simulink model "calc"  (R2021a)
settings: Solver=VariableStepAuto  StartTime=0.0  StopTime=10.0  RelTol=1e-3
undefined symbols (not defined in the file or in its folder): sigbuilder_block
settings Model: Creator=tomonori  LastModifiedBy=tomonori

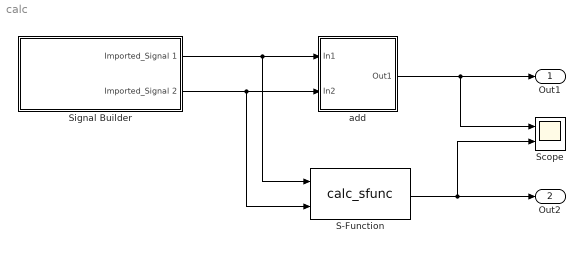
== system calc ==
  S-Function : S-Function  FunctionName=calc_sfunc  SFunctionDeploymentMode=off  EnableBusSupport=off
  Scope : Scope  NumInputPorts=2
  Signal Builder : Subsystem  Tag=STV Subsys  LoadFcn=sigbuilder_block('load',[4.5 187.5 550.5 387.75 ]);  StartFcn=sigbuilder_block('start');  StopFcn=sigbuilder_block('stop');  ClipboardFcn=sigbuilder_block('clipboard');  mask(Sigbuilder block){tuvar=[0:10]}
      mask help: Simulink:masks:SigbuilderBlock_MD
      mask init:
      | if ~strcmp(get_param(bdroot(gcbh),'SimulationStatus'),'stopped') tuvar = sigbuilder_block('maskInit'); end
      settings: CopyFcn=sigbuilder_block('copy');  DeleteFcn=sigbuilder_block('delete');  ModelCloseFcn=sigbuilder_block('modelClose');  PreSaveFcn=sigbuilder_block('preSave');  PauseFcn=sigbuilder_block('pause');  ContinueFcn=sigbuilder_block('continue');  NameChangeFcn=sigbuilder_block('namechange');  OpenFcn=sigbuilder_block('open',[4.5 187.5 550.5 387.75 ]);  CloseFcn=sigbuilder_block('close');
      mask Display: plot(0, 0, 100, 100,[2, 2, 32, 32, 2], [68, 8, 8, 68, 68],[32, 2], [38, 38], [32, 19, 2],[53, 60, 44], [32, 17, 17, 2],[16, 16, 31, 31]);txt = getActiveGroup(gcbh);text(2, 100, txt,'verticalAlignment', 'top');
  add : Subsystem
  Out1 : Outport
  Out2 : Outport  Port=2
  wires:
  Signal Builder/1(Imported_Signal 1) -> S-Function/1, add/1(In1)
  Signal Builder/2(Imported_Signal 2) -> S-Function/2, add/2(In2)
  add/1(Out1) -> Scope/1, Out1/1
  S-Function/1 -> Scope/2, Out2/1

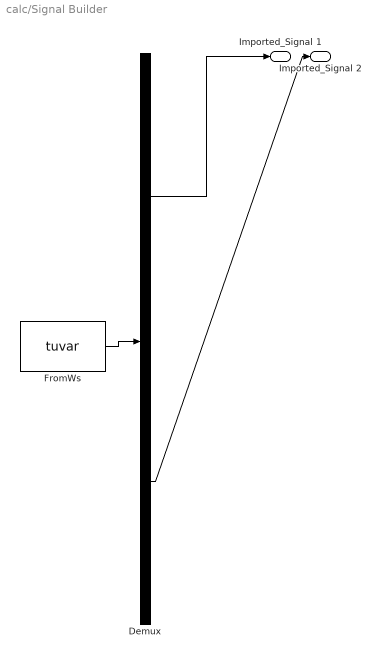
== system calc/Signal Builder ==
  Demux : Demux  Tag=STV Demux  Outputs=2
      settings: DisplayOption=none
  FromWs : FromWorkspace  Tag=STV FromWs  VariableName=tuvar
      SigBuilderData=|
      | common.afterFinalStr = 'Extrapolate'
      | common.sampleTime = 0
      | dataSet.timeRange = [1 10]
      | dataSet.name = 'Sheet1'
      | sbobj.Groups.Name = 'Sheet1'
      | sbobj.Groups.Signals(1).Name = 'Imported_Signal 1'
      | sbobj.Groups.Signals(1).XData = [1 2 3 4 5 6 7 8 9 10]
      | sbobj.Groups.Signals(1).YData = [2 3 4 5 6 6 7 7 8 8]
      | sbobj.Groups.Signals(2).Name = 'Imported_Signal 2'
      | sbobj.Groups.Signals(2).XData = [1 2 3 4 5 6 7 8 9 10]
      | sbobj.Groups.Signals(2).YData = [12 4 2 3 5 6 4 3 6 7]
      | sbobj.Groups.TimeRange = [1 10]
  Imported_Signal 1 : Outport  Tag=STV Outport
  Imported_Signal 2 : Outport  Tag=STV Outport  Port=2
  wires:
  Demux/1 -> Imported_Signal 1/1
  FromWs/1 -> Demux/1
  Demux/2 -> Imported_Signal 2/1

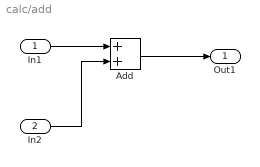
== system calc/add ==
  In1 : Inport
  In2 : Inport  Port=2
  Add : Sum
  Out1 : Outport
  wires:
  Add/1 -> Out1/1
  In2/1 -> Add/2
  In1/1 -> Add/1
